simulink model "openloop"  (Simulink 7.5)
settings: Solver=ode45  StartTime=0.0  StopTime=4  RelTol=1e-3
settings Model: Creator=iain  LastModifiedBy=iain

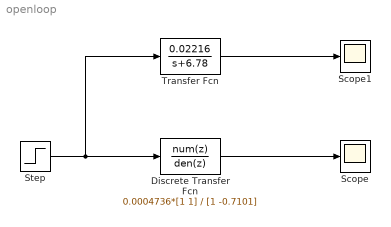
== system openloop ==
  Discrete Transfer Fcn : DiscreteTransferFcn  Numerator=0.0004736*[1 1]  Denominator=[1 -0.7101]  SampleTime=0.05
  Scope : Scope
  Scope1 : Scope
  Step : Step  SampleTime=0
  Transfer Fcn : TransferFcn  Numerator=[0.02216]  Denominator=[1 6.78]
  wires:
  Step/1 -> Discrete Transfer Fcn/1, Transfer Fcn/1
  Discrete Transfer Fcn/1 -> Scope/1
  Transfer Fcn/1 -> Scope1/1
